simulink model "cruise"  (R2017a)
settings: Solver=VariableStepAuto  StartTime=0.0  StopTime=10.0  RelTol=1e-3
values from neighbouring files (symbols this model uses):
  m = 50    [cruise_m.m]
settings Model: Creator=SHREYASH  LastModifiedBy=SHREYASH

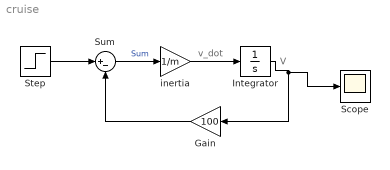
== system cruise ==
  note: V
  note: v_dot
  Gain : Gain  Gain=100
  Integrator : Integrator
  Scope : Scope
  Step : Step  SampleTime=0
  Sum : Sum  Inputs=|+-
  inertia : Gain  Gain=1/m
  wires:
  inertia/1 -> Integrator/1
  Integrator/1 -> Scope/1, Gain/1
  Sum/1 -> inertia/1  "Sum"
  Gain/1 -> Sum/2
  Step/1 -> Sum/1
